simulink model "nocontrol"  (R2020b)
settings: Solver=ode45  StartTime=0.0  StopTime=11658  RelTol=1e-5
values from neighbouring files (symbols this model uses):
  A = zeros(N_body+N_SP,1)    [main_detumbling.m]    (also in main_earthpointing.m; main_nocontrol.m)
  A_BN_0 = eye(3)    [main_detumbling.m]    (also in main_nocontrol.m)
  d = zeros(N_body+N_SP,3)    [main_detumbling.m]    (also in main_earthpointing.m; main_nocontrol.m)
  d_cg = [0.017 0 0]'    [main_detumbling.m]    (also in main_earthpointing.m; main_nocontrol.m)
  I = [Ix Iy Iz]    [main_detumbling.m]    (also in main_earthpointing.m; main_nocontrol.m)
  IGRF_coefficients = [1 1 2 2 2 3 3 3 3 4 4 4 ... (832 elements, 104x8)]    [IGRF_coefficients.mat]
  kep = [a; e; i; OM; om; theta]    [main_detumbling.m]    (also in main_earthpointing.m; main_nocontrol.m)
  N = zeros(N_body+N_SP,3)    [main_detumbling.m]    (also in main_earthpointing.m; main_nocontrol.m)
  theta = 0    [PlotEarth.m]    (also in main_detumbling.m = deg2rad(0); main_earthpointing.m = deg2rad(0); main_nocontrol.m = deg2rad(0))
  w_0 = deg2rad([8 13 4])    [main_detumbling.m]    (also in main_earthpointing.m = deg2rad([0 0 0]); main_nocontrol.m)
undefined symbols (not defined in the file or in its folder): IAU
libraries: aerolibtransform2 x1, aerolibconvert2 x1, dspmtrx3 x1
settings Model: Creator=GianMarco  LastModifiedBy=GianMarco

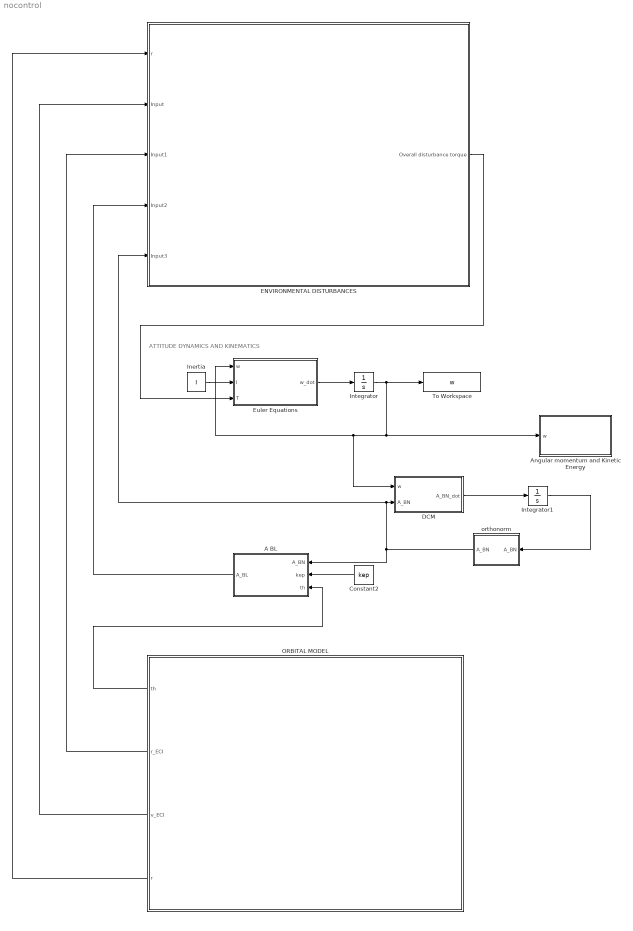
== system nocontrol ==
  note: ATTITUDE DYNAMICS AND KINEMATICS
  A BL : MATLAB Function  TreatAsAtomicUnit=on
  Angular momentum and Kinetic Energy : Subsystem
  Constant2 : Constant  Value=kep
  DCM : MATLAB Function  TreatAsAtomicUnit=on
  ENVIRONMENTAL DISTURBANCES : Subsystem
  Euler Equations : MATLAB Function  TreatAsAtomicUnit=on
  Inertia : Constant  Value=I
  Integrator : Integrator  InitialCondition=w_0
  Integrator1 : Integrator  InitialCondition=A_BN_0
  ORBITAL MODEL : Subsystem
  To Workspace : ToWorkspace  VariableName=w  SaveFormat=Timeseries  SampleTime=-1
  orthonorm : MATLAB Function  TreatAsAtomicUnit=on
  wires:
  Integrator/1 -> To Workspace/1, DCM/1(w), Euler Equations/1(w), Angular momentum and Kinetic Energy/1(w)
  Euler Equations/1(w_dot) -> Integrator/1
  Inertia/1 -> Euler Equations/2(I)
  DCM/1(A_BN_dot) -> Integrator1/1
  Integrator1/1 -> orthonorm/1("A_BN ")
  orthonorm/1(A_BN) -> ENVIRONMENTAL DISTURBANCES/5(Input3), DCM/2(A_BN), A BL/1(A_BN)
  Constant2/1 -> A BL/2(kep)
  ENVIRONMENTAL DISTURBANCES/1(Overall disturbance torque) -> Euler Equations/3(T)
  ORBITAL MODEL/2(r_ECI) -> ENVIRONMENTAL DISTURBANCES/3(Input1)
  ORBITAL MODEL/3(v_ECI) -> ENVIRONMENTAL DISTURBANCES/2(Input)
  ORBITAL MODEL/1(th) -> A BL/3(th)
  ORBITAL MODEL/4(r) -> ENVIRONMENTAL DISTURBANCES/1(r)
  A BL/1(A_BL) -> ENVIRONMENTAL DISTURBANCES/4(Input2)

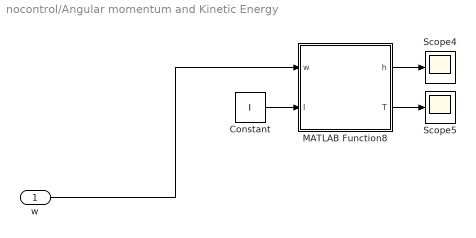
== system nocontrol/Angular momentum and Kinetic Energy ==
  w : Inport
  Constant : Constant  Value=I
  MATLAB Function8 : MATLAB Function  TreatAsAtomicUnit=on
  Scope4 : Scope
  Scope5 : Scope
  wires:
  MATLAB Function8/1(h) -> Scope4/1
  w/1 -> MATLAB Function8/1(w)
  MATLAB Function8/2(T) -> Scope5/1
  Constant/1 -> MATLAB Function8/2(I)

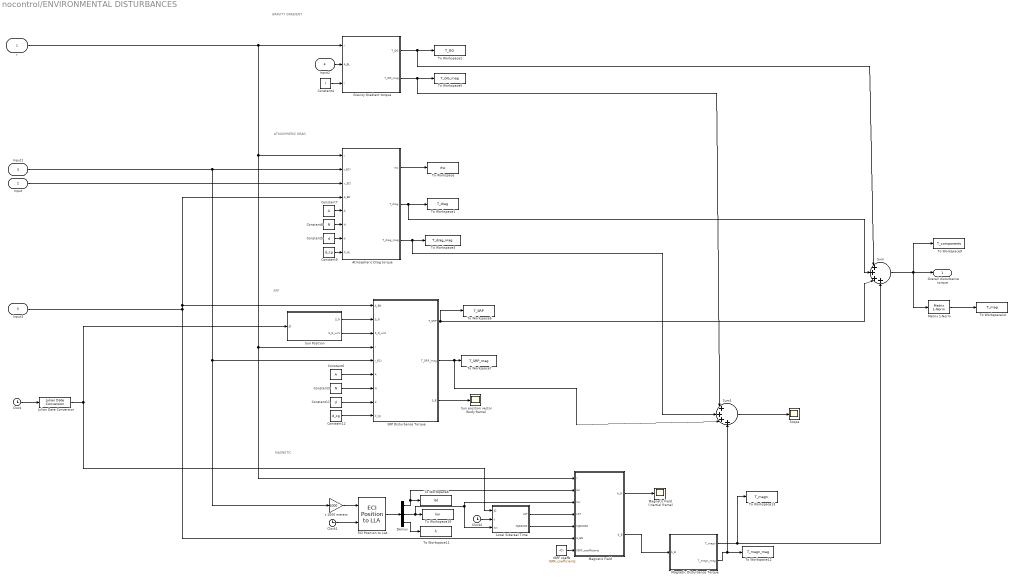
== system nocontrol/ENVIRONMENTAL DISTURBANCES ==
  note: MAGNETIC
  note: ATMOSPHERIC DRAG
  note: GRAVITY GRADIENT
  note: SRP
  r : Inport
  Input : Inport  Port=2
  Input1 : Inport  Port=3
  Input2 : Inport  Port=4
  Input3 : Inport  Port=5
  Atmospheric Drag torque : MATLAB Function  TreatAsAtomicUnit=on
  Clock : Clock
  Clock1 : Clock
  Clock2 : Clock
  Constant11 : Constant  Value=d
  Constant12 : Constant  Value=d_cg
  Constant3 : Constant  Value=N
  Constant4 : Constant  Value=I
  Constant5 : Constant  Value=d
  Constant6 : Constant  Value=A
  Constant7 : Constant  Value=A
  Constant8 : Constant  Value=N
  Constant9 : Constant  Value=d_cg
  Demux : Demux  Outputs=3
  ECI Position to LLA : aerolibtransform2/ECI Position to LLA  red=IAU-2000/2006  year=2022  month=January  day=1  hour=12  min=0  sec=0  deltaT=Sec  errorflag=Error  extraparamflag=off  eunits=Metric (MKS)  earthmodel=WGS84  flat=1/298.257223563  eqradius=6378137
      settings: AttributesFormatString=%<red>  SourceProductBaseCode=AE
  Gravity Gradient torque : MATLAB Function  TreatAsAtomicUnit=on
  IGRF coeffs : Constant  Value=IGRF_coefficients
  Julian Date Conversion : aerolibconvert2/Julian Date Conversion  year=2022  month=January  day=1  hour=12  min=0  sec=0  modflag=off  deltaT=Sec  errorflag=Error
      settings: SourceProductBaseCode=AE
  Local Sidereal Time : MATLAB Function  TreatAsAtomicUnit=on
  Magnetic Disturbance Torque : MATLAB Function  TreatAsAtomicUnit=on
  Magnetic Field : MATLAB Function  TreatAsAtomicUnit=on
  Magnetic Field (inertial frame) : Scope
  Matrix 1-Norm : dspmtrx3/Matrix  1-Norm  roundingMode=Floor  overflowMode=off  outputDataTypeStr=Inherit: Same as accumulator  outputMin=[]  outputMax=[]  outputLastDataTypeStr=Inherit: Same as accumulator
      settings: SourceProductBaseCode=DS
  SRP Disturbance Torque : MATLAB Function  TreatAsAtomicUnit=on
  Scope : Scope
  Sum : Sum  Inputs=|++++
  Sum1 : Sum  Inputs=|++++
  Sun Position : MATLAB Function  TreatAsAtomicUnit=on
  Sun position vector (body frame) : Scope
  To Workspace : ToWorkspace  VariableName=rho  SampleTime=-1
  To Workspace1 : ToWorkspace  VariableName=T_drag  SampleTime=-1
  To Workspace10 : ToWorkspace  VariableName=lon  SampleTime=-1
  To Workspace11 : ToWorkspace  VariableName=h  SampleTime=-1
  To Workspace12 : ToWorkspace  VariableName=T_magn_mag  SampleTime=-1
  To Workspace13 : ToWorkspace  VariableName=T_magn  SampleTime=-1
  To Workspace14 : ToWorkspace  VariableName=T_mag  SampleTime=-1
  To Workspace2 : ToWorkspace  VariableName=T_GG  SampleTime=-1
  To Workspace3 : ToWorkspace  VariableName=T_drag_mag  SampleTime=-1
  To Workspace5 : ToWorkspace  VariableName=T_GG_mag  SampleTime=-1
  To Workspace6 : ToWorkspace  VariableName=T_SRP  SampleTime=-1
  To Workspace7 : ToWorkspace  VariableName=T_SRP_mag  SampleTime=-1
  To Workspace8 : ToWorkspace  VariableName=lat  SampleTime=-1
  To Workspace9 : ToWorkspace  VariableName=T_components  SampleTime=-1
  x 1000 meters : Gain  Gain=1000
  Overall disturbance torque : Outport
  wires:
  Constant4/1 -> Gravity Gradient torque/3(I)
  Gravity Gradient torque/1(T_GG) -> Sum/1, To Workspace2/1
  Gravity Gradient torque/2(T_GG_mag) -> Sum1/1, To Workspace5/1
  Sun Position/1(S_N) -> SRP Disturbance Torque/2(S_N)
  Julian Date Conversion/1 -> Local Sidereal Time/1(JD), Sun Position/1(JD)
  Clock/1 -> Julian Date Conversion/1
  Constant3/1 -> SRP Disturbance Torque/7(N)
  Constant11/1 -> SRP Disturbance Torque/8(d)
  SRP Disturbance Torque/3(S_B) -> Sun position vector (body frame)/1
  Sun Position/2(S_N_unit) -> SRP Disturbance Torque/3(S_N_unit)
  SRP Disturbance Torque/2(T_SRP_mag) -> Sum1/3, To Workspace7/1
  Constant12/1 -> SRP Disturbance Torque/9(d_cg)
  SRP Disturbance Torque/1(T_SRP) -> Sum/3, To Workspace6/1
  Constant6/1 -> SRP Disturbance Torque/6(A)
  Magnetic Field/1(b_N) -> Magnetic Field (inertial frame)/1
  Magnetic Disturbance Torque/1(T_magn) -> To Workspace13/1, Sum/4
  Demux/2 -> To Workspace10/1, Local Sidereal Time/3(lon), Magnetic Field/3(lon)
  x 1000 meters/1 -> ECI Position to LLA/1
  Demux/1 -> Magnetic Field/2(lat), To Workspace8/1
  Clock2/1 -> Local Sidereal Time/2(t)
  Demux/3 -> To Workspace11/1
  IGRF coeffs/1 -> Magnetic Field/7(IGRF_coefficients)
  Clock1/1 -> ECI Position to LLA/2
  Magnetic Field/2(b_B) -> Magnetic Disturbance Torque/1(b_B)
  ECI Position to LLA/1 -> Demux/1
  Local Sidereal Time/1(LST) -> Magnetic Field/4(LST)
  Local Sidereal Time/2(MJD2000) -> Magnetic Field/5(MJD2000)
  Magnetic Disturbance Torque/2(T_magn_mag) -> Sum1/4, To Workspace12/1
  Constant7/1 -> Atmospheric Drag torque/5(A)
  Constant8/1 -> Atmospheric Drag torque/6(N)
  Constant5/1 -> Atmospheric Drag torque/7(d)
  Constant9/1 -> Atmospheric Drag torque/8(d_cg)
  Input/1 -> Atmospheric Drag torque/3(v_ECI)
  Input1/1 -> x 1000 meters/1, SRP Disturbance Torque/5(r_ECI), Atmospheric Drag torque/2(r_ECI)
  r/1 -> Atmospheric Drag torque/1(r), Magnetic Field/1(r), SRP Disturbance Torque/4(r), Gravity Gradient torque/1(r)
  Input2/1 -> Gravity Gradient torque/2(A_BL)
  Input3/1 -> Atmospheric Drag torque/4(A_BN), SRP Disturbance Torque/1(A_BN), Magnetic Field/6(A_BN)
  Atmospheric Drag torque/1(rho) -> To Workspace/1
  Atmospheric Drag torque/3(T_drag_mag) -> To Workspace3/1, Sum1/2
  Atmospheric Drag torque/2(T_drag) -> To Workspace1/1, Sum/2
  Sum/1 -> Matrix 1-Norm/1, Overall disturbance torque/1, To Workspace9/1
  Matrix 1-Norm/1 -> To Workspace14/1
  Sum1/1 -> Scope/1

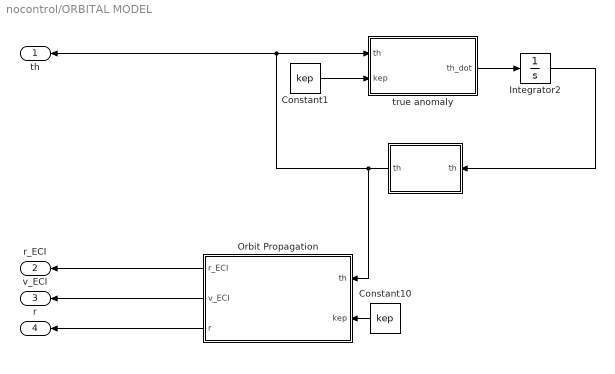
== system nocontrol/ORBITAL MODEL ==
  " " : MATLAB Function  TreatAsAtomicUnit=on
  Constant1 : Constant  Value=kep
  Constant10 : Constant  Value=kep
  Integrator2 : Integrator  InitialCondition=theta
  Orbit Propagation : MATLAB Function  TreatAsAtomicUnit=on
  true anomaly : MATLAB Function  TreatAsAtomicUnit=on
  th : Outport
  r_ECI : Outport  Port=2
  v_ECI : Outport  Port=3
  r : Outport  Port=4
  wires:
  Orbit Propagation/3(r) -> r/1
  Orbit Propagation/2(v_ECI) -> v_ECI/1
  Constant1/1 -> true anomaly/2(kep)
  Integrator2/1 -> " "/1("th ")
  true anomaly/1(th_dot) -> Integrator2/1
  Orbit Propagation/1(r_ECI) -> r_ECI/1
  Constant10/1 -> Orbit Propagation/2(kep)
  " "/1(th) -> Orbit Propagation/1(th), th/1, true anomaly/1(th)

== matlab function nocontrol/ENVIRONMENTAL DISTURBANCES/Gravity Gradient torque ==
  data: r input; T_GG output; A_BL input; I input; T_GG_mag output
function [T_GG,T_GG_mag]= GG(r,A_BL,I)

% Inertia moments of the 6U Cubesat with solar panels deployed [kg*m^2]
Ix=I(1);
Iy=I(2);
Iz=I(3);

%% GRAVITY GRADIENT TORQUE
% Gravitational constant and Earth's mass
G = 6.67408e-11; % [m^3*kg^-1*s^-2]
mt = 5.972e+24;  % [kg]

n = sqrt((3*G*mt)/(r*1e+3)^3);

% Direction cosines of the radial direction in principal axes
c = A_BL*[1 0 0]';

% GG disturbance torque [N*m]
T_GGx = (Iz-Iy)*n^2*c(3)*c(2);
T_GGy = (Ix-Iz)*n^2*c(1)*c(3);
T_GGz = (Iy-Ix)*n^2*c(2)*c(1);

T_GG = [T_GGx; T_GGy; T_GGz];

T_GG_mag = norm(T_GG);

== matlab function nocontrol/ENVIRONMENTAL DISTURBANCES/Atmospheric Drag torque ==
  data: r input; r_ECI input; v_ECI input; A_BN input; A input; N input; d input; d_cg input; rho output; T_drag output; T_drag_mag output
function [rho,T_drag,T_drag_mag]  = Drag(r,r_ECI,v_ECI,A_BN,A,N,d,d_cg)

%% Atmospheric density exponential model

% Earth radius
R_E = 6378.137; % [km]

% Altitude
h = r - R_E; % [km]

H = 0;
h0 = 0;
rho_0 = 0; 

if h > 200 && h <= 250
    H = 37.105;
    h0 = 200;
    rho_0 = 2.789e-10;
elseif h > 250 && h <= 300
    H = 45.546;
    h0 = 250;
    rho_0 = 7.248e-11;
elseif h > 300 && h <= 350
    H = 53.628;
    h0 = 300;
    rho_0 = 2.418e-11;
elseif h > 350 && h <= 400
    H = 53.298;
    h0 = 350;
    rho_0 = 9.158e-12;
elseif h > 400 && h <= 450
    H = 58.515;
    h0 = 400;
    rho_0 = 3.725e-12;
elseif h > 450 && h <= 500
    H = 60.828;
    h0 = 450;
    rho_0 = 1.585e-12;
elseif h > 500 && h <= 600
    H = 63.822;
    h0 = 500;
    rho_0 = 6.967e-13;
elseif h > 600 && h <= 700
    H = 71.835;
    h0 = 600;
    rho_0 = 1.454e-13;
elseif h > 700 && h <= 800
    H = 88.667;
    h0 = 700;
    rho_0 = 3.614e-14;
elseif h > 800 && h <= 900
    H = 124.64;
    h0 = 800;
    rho_0 = 1.170e-14;
elseif h > 900 && h < 1000
    H = 181.05;
    h0 = 900;
    rho_0 = 5.245e-15;
elseif h > 1000 
    H = 268.0;
    h0 = 1000;
    rho_0 = 3.019e-15;
end

rho = rho_0*exp(-(h-h0)/H); % [kg/m^3]


%% Atmospheric Drag Torque

% Earth's angular rate and radius: 
w_E = 2*pi/(23*3600 + 56*60 + 4.09); % [rad/s]

% Relative atmosphere velocity with respect to the inertial frame
v_rel_N = (v_ECI + cross([0 0 w_E]', r_ECI))*1000; % [m/s]

% Relative atmosphere velocity expressed in body frame
v_rel_B = (A_BN*v_rel_N);  % [m/s]
v_rel_B_unit = (v_rel_B/norm(v_rel_B));


% Number of sufaces considered
N_body = 6;
N_SP = 4;

% Drag coefficient
C_D = 2.2;

% Initialize vector
T_drag = zeros(3,1);

for k = 1:N_body+N_SP
    
    n_k = N(k,:)';
    
    if dot(n_k,v_rel_B_unit) > 0
        d_k = (d(k,:) - d_cg')';
        F_k = - 0.5 * C_D * rho * norm(v_rel_B)^2 * dot(n_k,v_rel_B_unit) * A(k) * v_rel_B_unit;
        T_drag_k = cross(d_k, F_k);
    else
        T_drag_k = zeros(3,1);
    end
    
    T_drag = T_drag + T_drag_k;
    
    T_drag_mag = norm(T_drag);
end

== matlab function nocontrol/ENVIRONMENTAL DISTURBANCES/SRP Disturbance Torque ==
  data: A_BN input; S_N input; S_N_unit input; T_SRP output; r input; r_ECI input; A input; N input; d input; d_cg input; T_SRP_mag output; S_B output
function [T_SRP, T_SRP_mag,S_B] = SRP(A_BN,S_N,S_N_unit,r,r_ECI,A,N,d,d_cg)

% Sun position vector with respect to body frame
S_B = A_BN*S_N;
S_B_norm = norm(S_B);
S_B_unit = S_B/S_B_norm;

% Earth radius [km]
R_E = 6378.137; 

% Shadow model
if dot(r_ECI,S_N_unit) < - sqrt(r^2 - R_E^2)
F  = 141.9; % [W/m^2]
else 
F = 1358 + 534.4 + 141.9; % [W/m^2] 
end

% Speed of light in vaccum [m/s]
c = 299792458; 

% Solar pressure
P = F/c;


% Number of surfaces considered
N_body = 6;
N_SP = 4;

% Specular and diffuse reflection coefficients
c_s_body = 0.5;     
c_d_body = 0.1;
c_s_SP = 0.8;
c_d_SP = 0.1;

% Compute SRP torque
T_SRP = zeros(3,1);

for k = 1:N_body+N_SP
    if k <= N_body
        c_s = c_s_body;     c_d = c_d_body;
    else
        c_s = c_s_SP;       c_d = c_d_SP;
    end
    
    n_k = N(k,:)';
    
    if dot(S_B_unit, n_k) > 0
        F_k = - P*A(k)*dot(S_B_unit,n_k) * ( (1-c_s)*S_B_unit + (2*c_s*dot(S_B_unit,n_k)+2/3*c_d)*n_k );
        d_k = (d(k,:) - d_cg')';
        T_SRP_k = cross(d_k, F_k);
    else
        T_SRP_k = zeros(3,1);
    end
    
    T_SRP = T_SRP + T_SRP_k;
    
        
end

T_SRP_mag = norm(T_SRP);

== matlab function nocontrol/ENVIRONMENTAL DISTURBANCES/Sun Position ==
  data: S_N output; JD input; S_N_unit output
function [S_N,S_N_unit] = SunPosition(JD)

% From Markley, Crassidis: Fundamentals of Spacecraft Attitude
% Determination & Control (2014), pag. 420-422.

% Time T_0 in Julian centuries between the Julian day JD and J2000
T_0 = (JD - 2451545)/36525;

% Sun's Mean Longitude and Mean Anomaly [deg]
phi_sun = 280.460 + 36000.771*T_0;

M_sun = 357.5277233 + 35999.05034*T_0;

% Wrap to 360° 
if (phi_sun >= 360)
phi_sun = phi_sun - fix(phi_sun/360)*360; 
elseif (phi_sun < 0)
phi_sun = phi_sun - (fix(phi_sun/360) - 1)*360; 
end

if (M_sun >= 360)
M_sun = M_sun - fix(M_sun/360)*360; 
elseif (M_sun < 0)
M_sun = M_sun - (fix(M_sun/360) - 1)*360; 
end

% Ecliptic longitude 
phi_ecl = phi_sun + 1.914666471*sind(M_sun) + 0.019994643*sind(2*M_sun);

% Obliquity of the ecliptic
eps_ecl = 23.439291 - 0.0130042*T_0;

% Unit vector in the direction from Earth to Sun
S_N_unit = [cosd(phi_ecl); cosd(eps_ecl)*sind(phi_ecl); sind(eps_ecl)*sind(phi_ecl)];

% Distance between the Earth and the Sun [AU]
R_S = 1.000140612 - 0.016708617*cosd(M_sun) - 0.000139589*cosd(2*M_sun);

% Position vector from the Earth to the Sun 
S_N = R_S*S_N_unit; % [AU]

S_N = S_N*149597870.691; % [km]

== matlab function nocontrol/ENVIRONMENTAL DISTURBANCES/Local Sidereal Time ==
  data: JD input; LST output; t input; lon input; MJD2000 output
function [LST,MJD2000] = LST(JD,t,lon)

% Adapted from: H.D. Curtis: Orbital Mechanics for Engineering Students
% (2014), pag.261. 

% Time T_0 in Julian centuries between the Julian day JD and J2000
T_0 = (JD - 2451545)/36525;

% Modified Julian Date
MJD2000 = JD - 2400000.5 - 51544.5;

% Greenwich sidereal time at 0 h UT
theta_G0 = 100.4606184 + 36000.77004*T_0 + 0.000387933*T_0^2 - 2.583e-8*T_0^3;

% Reduce theta_G0 so it lies in the range 0 - 360 degrees
if (theta_G0 >= 360)
theta_G0 = theta_G0 - fix(theta_G0/360)*360; 
elseif (theta_G0 < 0)
theta_G0 = theta_G0 - (fix(theta_G0/360) - 1)*360; 
end

% Universal Time (UT) in hours 
UT_0 = 12;
UT = UT_0 + t/3600;

% Greenwich sidereal time
theta_G = theta_G0 + 360.98564724*UT/24;

% Local sidereal time
LST = theta_G + lon;

% Reduce LST to the range 0 - 360 degrees:
LST = LST - 360*fix(LST/360);

== matlab function nocontrol/ENVIRONMENTAL DISTURBANCES/Magnetic Field ==
  data: r input; b_N output; lat input; lon input; LST input; MJD2000 input; A_BN input; b_B output; IGRF_coefficients input
function [b_N,b_B] = MagneticField(r,lat,lon,LST,MJD2000,A_BN,IGRF_coefficients)

% Geocentric radius in [m]
r = r*10^3;

% Compute colatitude and longitude in radians
colat=(90-lat)*pi/180;
lon = lon*pi/180;

% Reference radius used in IGRF [m]
R_E = 6371.2*10^3; 

% Read in the g and h Schmidt quasi-normalized coefficients from .mat file
gn = IGRF_coefficients(:,1);
gm = IGRF_coefficients(:,2);
gvali = IGRF_coefficients(:,3);
gsvi = IGRF_coefficients(:,4);
hn = IGRF_coefficients(:,5);
hm = IGRF_coefficients(:,6);
hvali = IGRF_coefficients(:,7);
hsvi = IGRF_coefficients(:,8);

% Set the IGRF order
N = 13;
g = zeros(N,N+1);
h = zeros(N,N+1);

for x=1:length(gn)
    g(gn(x),gm(x)+1) = gvali(x) + gsvi(x)*MJD2000/365;
    h(hn(x),hm(x)+1) = hvali(x) + hsvi(x)*MJD2000/365;
end

% Initialize the variables:
% B_r    B in the radial direction
% B_th   B in the theta direction
% B_phi  B in the phi direction
% P      Associated Legendre polynomial evaluated at cos(theta)
%        The nomenclature for the recursive values generally follows
%        the form P10 = P(n-1,m-0)
% dP     Partial derivative of P with respect to theta

B_r = 0; B_th = 0; B_phi = 0;
P11 = 1; P10 = P11;
dP11 = 0; dP10 = dP11;
P20 = 0; dP20 = 0;

% Compute the magnetic field strenght in local tangential coordinates with
% recursive formulas
for m=0:N
    for n=1:N
        if m<=n
            % Compute the Legendre polynomials and their derivatives
            if n == m
                P2 = sin(colat)*P11;
                dP2 = sin(colat)*dP11 + cos(colat)*P11;
                P11 = P2; P10 = P11; P20 = 0;
                dP11 = dP2; dP10 = dP11; dP20 = 0;
            elseif n == 1
                P2 = cos(colat)*P10;
                dP2 = cos(colat)*dP10 - sin(colat)*P10;
                P20 = P10; P10 = P2;
                dP20 = dP10; dP10 = dP2;
            else
                K = ((n-1)^2-m^2)/((2*n-1)*(2*n-3));
                P2 = cos(colat)*P10 - K*P20;
                dP2 = cos(colat)*dP10 - sin(colat)*P10 - K*dP20;
                P20 = P10; P10 = P2;
                dP20 = dP10; dP10 = dP2;
            end
            
            % Calculate B_r, B_th, and B_phi
            B_r = B_r + (R_E/r)^(n+2)*(n+1)*...
                ((g(n,m+1)*cos(m*lon) + h(n,m+1)*sin(m*lon))*P2);
            B_th = B_th + (R_E/r)^(n+2)*...
                ((g(n,m+1)*cos(m*lon) + h(n,m+1)*sin(m*lon))*dP2);
            B_phi = B_phi + (R_E/r)^(n+2)*...
                (m*(-g(n,m+1)*sin(m*lon) + h(n,m+1)*cos(m*lon))* P2);
        end
    end
end

B_th = -B_th;
B_phi = -B_phi/sin(colat);

% Convert latitude and LST from degrees to radians
lat = lat*pi/180;
LST = LST*pi/180;

% Convert B_r, B_th, B_phi from tangential spherical to ECI coordinates
B_x = (B_r*cos(lat)+B_th*sin(lat))*cos(LST) - B_phi*sin(LST);
B_y = (B_r*cos(lat)+B_th*sin(lat))*sin(LST) + B_phi*cos(LST);
B_z = (B_r*sin(lat)-B_th*cos(lat));

% Compute the Magnetic Field Vector in Tesla
b_N = [B_x; B_y; B_z]*1e-9;

b_B = A_BN*b_N;

== matlab function nocontrol/ENVIRONMENTAL DISTURBANCES/Magnetic Disturbance Torque ==
  data: b_B input; T_magn output; T_magn_mag output
function [T_magn,T_magn_mag] = Magnetic(b_B)

% Residual magnetic induction due to currents in the satellite [N*m/T]
m = [0.1; 0.1; 0.1];

% Magnetic disturbance torque [N*m]
T_magn = cross(m,b_B);

T_magn_mag = norm(T_magn);

== matlab function nocontrol/Euler Equations ==
  data: w input; I input; w_dot output; T input
function w_dot = Euler_Equations(w,I,T)

% Inertia moments of the 6U Cubesat with solar panels deployed [kg*m^2]
Ix = I(1);
Iy = I(2);
Iz = I(3);

Kx=(Iy-Iz)/Ix;
Ky=(Iz-Ix)/Iy;
Kz=(Ix-Iy)/Iz;

% Euler Equations
w_dot = zeros(3,1);
w_dot(1)=Kx*w(2)*w(3) + T(1)/Ix;
w_dot(2)=Ky*w(1)*w(3) + T(2)/Iy;
w_dot(3)=Kz*w(1)*w(2) + T(3)/Iz;

== matlab function nocontrol/DCM ==
  data: w input; A_BN_dot output; A_BN input
function A_BN_dot = DCM(w,A_BN)

W_cross = [0,    -w(3),  w(2);
           w(3),   0,   -w(1);
          -w(2),  w(1),   0];


A_BN_dot = -W_cross * A_BN;

== matlab function nocontrol/orthonorm ==
  data: A_BN input; A_BN output
function A_BN = orthonorm(A_BN)

for k=1:3
A_BN=3/2 * A_BN - 1/2 * A_BN*A_BN'*A_BN;
end

== matlab function nocontrol/ORBITAL MODEL/true anomaly ==
  data: th input; th_dot output; kep input
function th_dot = true_anomaly(th,kep)

% Semi-major axis [km] and eccentricity [-]
a = kep(1);
e = kep(2);

% Set Earth's standard gravitational parameter [km^3/s^2]
mu_E = 398600;  

% Orbital mean motion [rad/s]
n = sqrt(mu_E/a^3);  

% True anomaly derivative
th_dot = (n*(1+e*cos(th))^2)/((1-e^2)^(3/2));

== matlab function nocontrol/A BL ==
  data: A_BN input; kep input; th input; A_BL output
function A_BL = fcn(A_BN,kep,th)

% Inclination [rad], RAAN [rad] and Argument of perigee [rad]
i = kep(3);   
OM = kep(4);  
om = kep(5);  

% Rotation matrices
R3_omth = [cos(om+th) sin(om+th) 0; -sin(om+th) cos(om+th) 0; 0 0 1];
R1_i = [1 0 0; 0 cos(i) sin(i); 0 -sin(i) cos(i)];
R3_OM = [cos(OM) sin(OM) 0; -sin(OM) cos(OM) 0; 0 0 1];

% Rotation matrix Inertial frame --> LVLH
A_LN = R3_omth*R1_i*R3_OM;

% Rotation matrix LVLH --> Body frame
A_BL = A_BN*A_LN';

== matlab function nocontrol/ORBITAL MODEL/  ==
  data: th input; th output
function th = wrapto2pi(th)

% Wrap true anomaly between 0 and 2pi.

if th < 2*pi
    th=th;
else
    th=th-2*pi;
end
end

== matlab function nocontrol/ORBITAL MODEL/Orbit Propagation ==
  data: th input; r_ECI output; kep input; v_ECI output; r output
function [r_ECI,v_ECI,r] = OrbitPropagation(th,kep)

% Orbital parameters
a = kep(1);
e = kep(2);
i = kep(3);
OM = kep(4);
om = kep(5);

% Semilatus rectum [km]
p = a*(1-e^2);

% Orbital radius [km]
r = p/(1+e*cos(th)); 

% Earth's standard gravitational parameter [km^3/s^2]
mu_E = 398600; 

% Rotation matrices: Earth-Centered Inertial --> Perifocal (ECI --> PF)
R_om = [cos(om)  sin(om)    0   ;
        -sin(om) cos(om)    0   ;
           0        0       1   ];
       
R_i  = [   1        0       0   ;
           0     cos(i)   sin(i);
           0    -sin(i)   cos(i)];
       
R_OM = [cos(OM)  sin(OM)    0   ;
        -sin(OM) cos(OM)    0   ;
           0        0       1   ];
    
R313 = R_om * R_i * R_OM; 

% Position and velocity vectors in perifocal coordinates
r_PF = r * [cos(th), sin(th), 0]';
v_PF = sqrt(mu_E/p) * [-sin(th), (e+cos(th)), 0]';

% PF --> ECI transformation
r_ECI = R313'* r_PF;
v_ECI = R313'* v_PF;

== matlab function nocontrol/Angular momentum and Kinetic Energy/MATLAB Function8 ==
  data: w input; h output; T output; I input
function [h,T] = fcn(w,I)


Ix = I(1);
Iy = I(2);
Iz = I(3);

w_x=w(1);
w_y=w(2);
w_z=w(3); 

h=sqrt( (Ix*w_x)^2 + (Iy*w_y)^2 + (Iz*w_z)^2 );

T=Ix*w_x^2 + Iy*w_y^2 + Iz*w_z^2;
